simulink model "HIL_SS"  (Simulink 7.2)
settings: Solver=ode4  StartTime=0.0  StopTime=inf  FixedStep=0.002  RelTol=1e-3
PostLoadFcn:
  | qc_set_target_type(getConfigSet(bdroot, 'QUARC Default Target Configuration'));
values from neighbouring files (symbols this model uses):
  A = [-4 -0.03; 0.75 -10]    [MDLsisotool.m]    (also in dadosSS.mat = [-31.7887619239  -14.7359524048; 16  0])
  B = [2; 0]    [MDLsisotool.m]    (also in dadosSS.mat = [16 0])
  C = [0 1]    [MDLsisotool.m]    (also in dadosSS.mat = [0 22.1495321335])
  D = 0    [MDLsisotool.m]    (also in dadosSS.mat)
  Ki = Kext(3)    [MDLsspace.m]    (also in dadosSS.mat = -0.0370352066606; ssGera.m)
  Kproc = [Kext(1), Kext(2)]    [MDLsspace.m]    (also in dadosSS.mat = [-0.861797620241 -0.503028275301]; ssGera.m)
  L = (acker(A', C', polosObs))'    [MDLsspace.m]    (also in dadosSS.mat = [-0.306409103952 0.415866033676]; ssGera.m)
undefined symbols (not defined in the file or in its folder): HIL
libraries: quarc_library x3, simulink x1, simulink_extras x1
settings Model: Creator=pmartin  LastModifiedBy=aluno  SimulationMode=external  ExtModeTrigDuration=5000
settings SolverCC: PositivePriorityOrder=on
settings OptimizationCC: InitFltsAndDblsToZero=on
settings DebuggingCC: SaveWithParameterizedLinksMsg=none  MultiTaskDSMMsg=warning  MultiTaskCondExecSysMsg=none  StrictBusMsg=None
settings RTWCC: SystemTargetFile=quarc_windows.tlc  TemplateMakefile=quarc_default_tmf  Description=QUARC Win32 Target  ProcessScript=quarc_windows_make_rtw_hook
settings STFCustomTargetCC: TargetPreCompLibLocation=C:\DOCUME~1\ALLUSE~1\DADOSD~1\QUARC\lib\2008b\windows\release  SystemTargetFile=quarc_windows.tlc
settings GRTTargetCC: TargetPreCompLibLocation=C:\DOCUME~1\ALLUSE~1\DADOSD~1\QUARC\lib\2008b\windows\release  CompOptLevelCompliant=off  MatFileLogging=off  ExtMode=on  ExtModeMexFile=quarc_comm

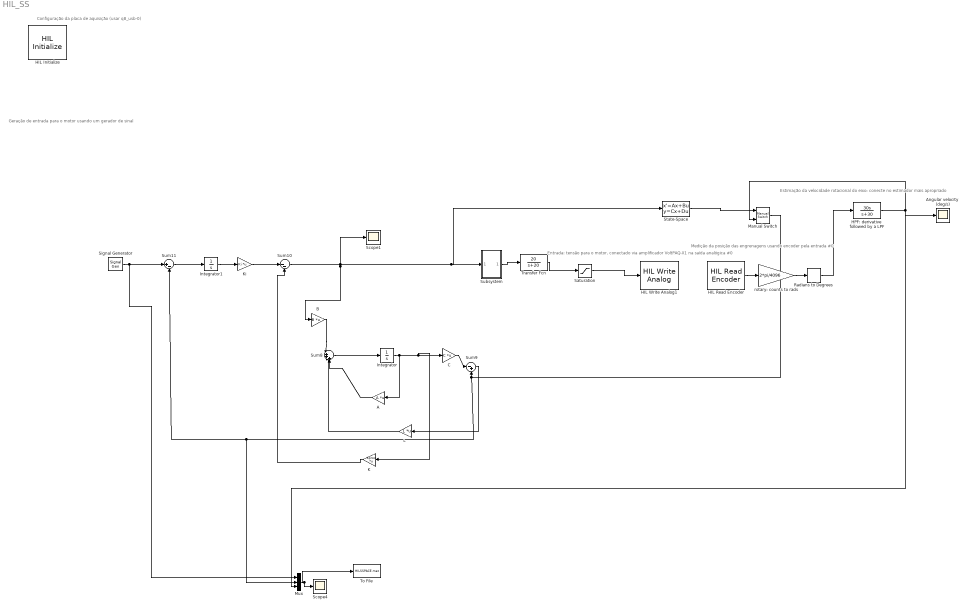
== system HIL_SS ==
  note: Medição da posição das engrenagens usando
      | encoder pela entrada #0
  note: Configuração da placa de aquisição (usar q8_usb-0)
  note: Entrada: tensão para o motor, conectado via
      | amplificador VoltPAQ-X1 na saída analógica #0
  note: Geração de entrada para o motor
      | usando um gerador de sinal
  note: Estimação da velocidade rotacional do eixo:
      | conecte no estimador mais apropriado
  A : Gain  Orientation=left  Gain=A  Multiplication=Matrix(K*u)
  Angular velocity  (deg/s) : Scope
      settings: TickLabels=on  TimeRange=10  YMin=-100  YMax=125  SaveName=data_xc1  DataFormat=Array
  B : Gain  Gain=B  Multiplication=Matrix(K*u)
  C : Gain  Gain=C  Multiplication=Matrix(K*u)
  HIL Initialize : quarc_library/Data Acquisition/Generic/Configuration/HIL Initialize  object_name=HIL-1  board_type=q8_usb  board_number=0  board_options=update_rate=normal  exclusive=off  active=off  hardware_clocks=[0:2]  clock_modes=[]  set_clock_params_at_start=off  set_clock_params_at_switch_in=off  analog_input_channels=[0:7]  analog_input_maximums=10  analog_input_minimums=-10  set_analog_input_params_at_start=on  set_analog_input_params_at_switch_in=off  analog_output_channels=[0:7]  analog_output_maximums=10  analog_output_minimums=-10  initial_analog_outputs=[0]  final_analog_outputs=[0]  watchdog_analog_outputs=0  set_analog_output_params_at_start=on  set_analog_output_params_at_switch_in=off  set_analog_outputs_at_start=on  set_analog_outputs_at_switch_in=off  set_analog_outputs_at_terminate=on  set_analog_outputs_at_switch_out=off  set_analog_outputs_on_watchdog=off  digital_input_channels=[]  digital_output_channels=[0:7]  digital_output_configuration=[]  initial_digital_outputs=[0]  final_digital_outputs=[0]  watchdog_digital_outputs=[0]  set_digital_output_params_at_start=off  set_digital_output_params_at_switch_in=off  set_digital_outputs_at_start=on  set_digital_outputs_at_switch_in=off  set_digital_outputs_at_terminate=on  set_digital_outputs_at_switch_out=off  set_digital_outputs_on_watchdog=off  encoder_channels=[0:7]  quadrature=[4]  encoder_filter_frequency=[]  initial_encoder_counts=[0]  set_encoder_params_at_start=on  set_encoder_params_at_switch_in=off  set_encoder_counts_at_start=on  set_encoder_counts_at_switch_in=off  pwm_channels=[0:7]  pwm_modes=0  pwm_frequency=99.532799999999995e6/4095  pwm_configuration=[0]  pwm_alignment=[0]  pwm_polarity=[1]  pwm_leading_deadband=[0]  pwm_trailing_deadband=[0]  initial_pwm_outputs=[0]  final_pwm_outputs=[0]  watchdog_pwm_outputs=[0]  set_pwm_params_at_start=on  set_pwm_params_at_switch_in=off  set_pwm_outputs_at_start=on  set_pwm_outputs_at_switch_in=off  set_pwm_outputs_at_terminate=on  set_pwm_outputs_at_switch_out=off  set_pwm_outputs_on_watchdog=off  other_output_channels=[]  initial_other_outputs=[]  final_other_outputs=[]  watchdog_other_outputs=[]  set_other_outputs_at_start=off  set_other_outputs_at_switch_in=off  set_other_outputs_at_terminate=off  set_other_outputs_at_switch_out=off  set_other_outputs_on_watchdog=off
  HIL Read Encoder : quarc_library/Data Acquisition/Generic/Immediate I//O/HIL Read Encoder  object_name=HIL-1  channels=[0]  sample_time=qc_get_step_size  active=on  vector_output=off  data_type_mode=Inherit via back propagation  data_type=double
  HIL Write Analog1 : quarc_library/Data Acquisition/Generic/Immediate I//O/HIL Write Analog  object_name=HIL-1  channels=0  sample_time=-1  active=off  vector_input=off
  HPF: derivative  followed by a LPF : TransferFcn  Numerator=[30 0]  Denominator=[1 30]
  Integrator : Integrator
  Integrator1 : Integrator
  K : Gain  Orientation=left  Gain=Kproc  Multiplication=Matrix(K*u)
  Ki : Gain  Gain=Ki  Multiplication=Matrix(K*u)
  L : Gain  Orientation=left  Gain=L  Multiplication=Matrix(K*u)
  Manual Switch : simulink/Signal Routing/Manual Switch  SystemSampleTime=-1  sw=0  action=0  varsize=off
  Mux : Mux  Inputs=3
  Radians to Degrees : simulink_extras/Transformations/Radians to Degrees  SystemSampleTime=-1
  Saturation : Saturate  UpperLimit=10  LowerLimit=-10  OutDataType=sfix(16)  OutScaling=2^0
  Scope1 : Scope
      settings: YMin=-1.25e+308  YMax=0
  Scope4 : Scope
      settings: YMin=-50  YMax=50  SaveName=ScopeData4
  Signal Generator : SignalGenerator  WaveForm=square  Amplitude=45  Frequency=1/5
  State-Space : StateSpace  A=A  B=B  C=C  D=D
  Subsystem : Subsystem
  Sum10 : Sum  Inputs=|--
  Sum11 : Sum  Inputs=|+-
  Sum8 : Sum  Inputs=|+++
  Sum9 : Sum  Inputs=|-+
  To File : ToFile  Filename=HILSSPACE.mat
  Transfer Fcn : TransferFcn  Numerator=[20]  Denominator=[1, 20]
  rotary: counts to rads : Gain  Gain=2*pi/4096  SaturateOnIntegerOverflow=on  OutDataTypeStr=Inherit: Same as input  ParamDataTypeStr=Inherit: Same as input
  wires:
  HIL Read Encoder/1 -> rotary: counts to rads/1
  rotary: counts to rads/1 -> Radians to Degrees/1
  HPF: derivative  followed by a LPF/1 -> Angular velocity  (deg/s)/1, Manual Switch/2, Mux/3
  Radians to Degrees/1 -> HPF: derivative  followed by a LPF/1
  Saturation/1 -> HIL Write Analog1/1
  Sum10/1 -> B/1, Scope1/1, State-Space/1, Subsystem/1(In1)
  Sum8/1 -> Integrator/1
  Integrator/1 -> A/1, C/1, K/1
  A/1 -> Sum8/3
  C/1 -> Sum9/1
  B/1 -> Sum8/1
  Sum9/1 -> L/1
  L/1 -> Sum8/2
  Integrator1/1 -> Ki/1
  Ki/1 -> Sum10/1
  Sum11/1 -> Integrator1/1
  Signal Generator/1 -> Sum11/1, Mux/1
  Mux/1 -> Scope4/1, To File/1
  K/1 -> Sum10/2
  Transfer Fcn/1 -> Saturation/1
  State-Space/1 -> Manual Switch/1
  Manual Switch/1 -> Sum9/2, Sum11/2, Mux/2
  Subsystem/1(Out1) -> Transfer Fcn/1

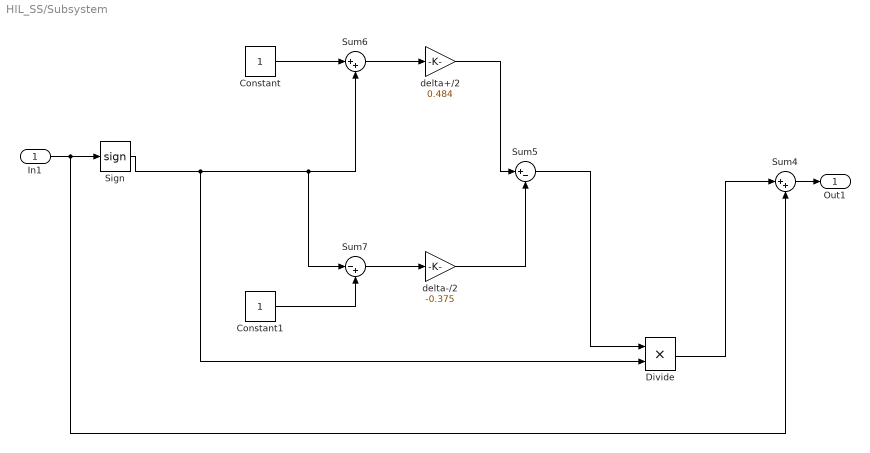
== system HIL_SS/Subsystem ==
  In1 : Inport
  Constant : Constant
  Constant1 : Constant
  Divide : Product  Inputs=**
  Sign : Signum
  Sum4 : Sum  Inputs=|++
  Sum5 : Sum  Inputs=|+-
  Sum6 : Sum  Inputs=|++
  Sum7 : Sum  Inputs=|-+
  delta+/2 : Gain  Gain=0.484
  delta-/2 : Gain  Gain=-0.375
  Out1 : Outport
  wires:
  Sign/1 -> Divide/2, Sum7/1, Sum6/2
  Sum6/1 -> delta+/2/1
  Sum7/1 -> delta-/2/1
  delta-/2/1 -> Sum5/2
  delta+/2/1 -> Sum5/1
  Sum5/1 -> Divide/1
  Divide/1 -> Sum4/1
  Constant1/1 -> Sum7/2
  Constant/1 -> Sum6/1
  In1/1 -> Sum4/2, Sign/1
  Sum4/1 -> Out1/1
